simulink model "Puma"  (R2018b)
settings: Solver=VariableStepAuto  StartTime=0.0  StopTime=2  RelTol=1e-3
values from neighbouring files (symbols this model uses):
  Bm = 0.01    [Run.m]
  Kb = 7.5    [Run.m]
  Km = 7.5    [Run.m]
  m1d = m1*d/(h+d)    (= 0.375)    [Run.m]
  m1h = m1*h/(h+d)    (= 1.625)    [Run.m]
  r = 50    [Run.m]
  Ra = 50    [Run.m]
  th1_0 = 0    [Run.m]
  th2_0 = 0    [Run.m]
  th3_0 = 0    [Run.m]
  Va1 = Va    (= 48)    [Run.m]
  Va2 = Va    (= 48)    [Run.m]
  Va3 = Va    (= 48)    [Run.m]
libraries: nesl_utility x13, sm_lib x11
settings Model: Creator=Erfan Etesami  LastModifiedBy=Erfan Etesami

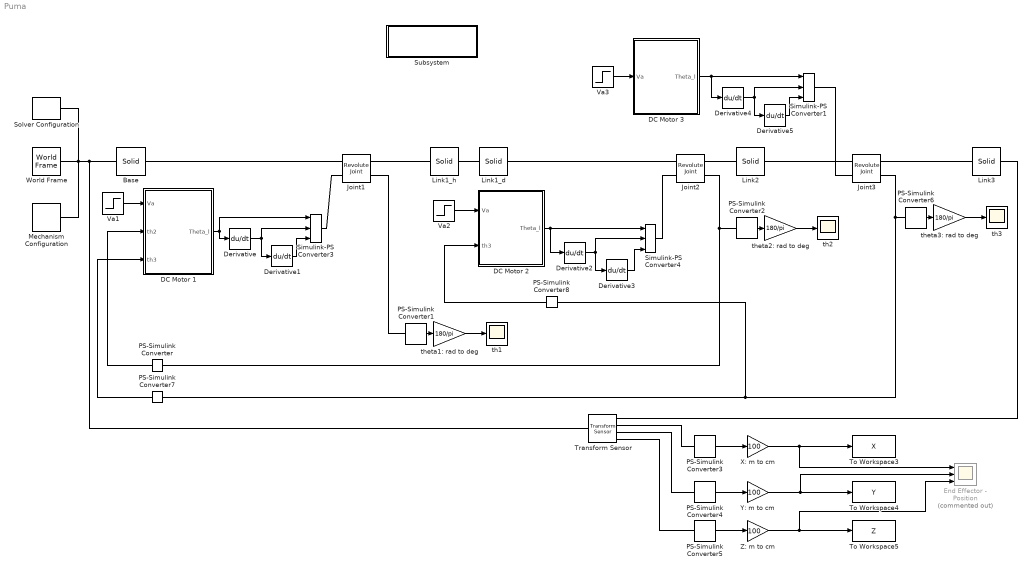
== system Puma ==
  Base : sm_lib/Body Elements/Solid  InertiaType=CalculateFromGeometry  Mass=1  MassUnits=kg  CenterOfMass=[0 0 0]  CenterOfMassUnits=m  MomentsOfInertia=[1 1 1]  MomentsOfInertiaUnits=kg*m^2  ProductsOfInertia=[0 0 0]  ProductsOfInertiaUnits=kg*m^2  BasedOnType=Density  Density=1000  DensityUnits=kg/m^3  DoExposeReferenceFrame=off  SerializedFrames=<Frames><Frame><Id>Frame1</Id><Value><Name>F0</Name><Origin><Source>GeometricFeature</Source><FeatureName>bottom surface</FeatureName></Origin><PrimaryAxis><DefinedDirection>+Y</DefinedDirection><Source>ReferenceFrame</Source><SourceDirection>+Z</SourceDirection><FeatureName></FeatureName></PrimaryAxis><SecondaryAxis><DefinedDirection>+X</DefinedDirection><Source>ReferenceFrame</Source><SourceDirection>+X</SourceDirection><FeatureName></FeatureName></SecondaryAxis></Value></Frame><Frame><Id>Frame2</Id><Value><Name>Ft</Name><Origin><Source>GeometricFeature</Source><FeatureName>bottom surface</FeatureName></Origin><PrimaryAxis><DefinedDirection>+Z</DefinedDirection><Source>ReferenceFrame</Source><SourceDirection>+Z</SourceDirection><FeatureName></FeatureName></PrimaryAxis><SecondaryAxis><DefinedDirection>+X</DefinedDirection><Source>ReferenceFrame</Source><SourceDirection>+X</SourceDirection><FeatureName></FeatureName></SecondaryAxis></Value></Frame></Frames>  GraphicType=FromGeometry  MarkerShape=Sphere  MarkerSize=10  GraphicVisPropType=SimpleVisualProperties  GraphicDiffuseColor=[0.5 0.5 0.5]  GraphicSpecularColor=[0.5 0.5 0.5 1.0]  GraphicAmbientColor=[0.15 0.15 0.15 1.0]  GraphicEmissiveColor=[0.0 0.0 0.0 1.0]  GraphicShininess=75  GraphicOpacity=1.0  GeometryShape=Cylinder  RectangleSize=[1 1]  RectangleSizeUnits=m  BrickDimensions=[1 1 65]  BrickDimensionUnits=cm  CylinderRadius=10  CylinderRadiusUnits=cm  CylinderLength=5  CylinderLengthUnits=cm  SphereRadius=1  SphereRadiusUnits=m  EllipsoidRadii=[1 1 1]  EllipsoidRadiiUnits=m  ExtrusionCrossSection=[1 1; -1 1; -1 -1; 1 -1]  ExtrusionCrossSectionUnits=m  ExtrusionLength=1  ExtrusionLengthUnits=m  PolygonNumSides=3  PolygonOuterRadius=1  PolygonOuterRadiusUnits=m  ExtGeomFileType=STEP  ExtGeomFileUnits=m  RevolutionCrossSection=[1 1; 1 -1; 2 -1; 2 1]  RevolutionCrossSectionUnits=m  RevolutionExtent=Full  RevolutionAngle=180  RevolutionAngleUnits=deg
  DC Motor 1 : Subsystem
  DC Motor 2 : Subsystem
  DC Motor 3 : Subsystem
  Derivative{,1..5} (6 alike) : Derivative
  End Effector - Position : Scope  Commented=on  NumInputPorts=3
  Joint1 : sm_lib/Joints/Revolute Joint  SenseConstraintForce=off  SenseConstraintForceX=off  SenseConstraintForceY=off  SenseConstraintForceZ=off  SenseConstraintTorque=off  SenseConstraintTorqueX=off  SenseConstraintTorqueY=off  SenseConstraintTorqueZ=off  SenseTotalForce=off  SenseTotalForceX=off  SenseTotalForceY=off  SenseTotalForceZ=off  SenseTotalTorque=off  SenseTotalTorqueX=off  SenseTotalTorqueY=off  SenseTotalTorqueZ=off  CompositeWrenchDir=FollowerOnBase  CompositeWrenchFrame=BaseFrame  EquilibriumPosition=0  EquilibriumPositionUnits=deg  SpringStiffness=0  SpringStiffnessUnits=N*m/deg  DampingCoefficient=0  DampingCoefficientUnits=N*m/(deg/s)  TorqueActuationMode=ComputedTorque  MotionActuationMode=InputMotion  SensePosition=on  SenseVelocity=off  SenseAcceleration=off  SenseTorqueForce=off  PositionTargetSpecify=off  PositionTargetPriority=High  PositionTargetValue=0  PositionTargetValueUnits=deg  VelocityTargetSpecify=off  VelocityTargetPriority=High  VelocityTargetValue=0  VelocityTargetValueUnits=deg/s
  Joint2 : sm_lib/Joints/Revolute Joint  SenseConstraintForce=off  SenseConstraintForceX=off  SenseConstraintForceY=off  SenseConstraintForceZ=off  SenseConstraintTorque=off  SenseConstraintTorqueX=off  SenseConstraintTorqueY=off  SenseConstraintTorqueZ=off  SenseTotalForce=off  SenseTotalForceX=off  SenseTotalForceY=off  SenseTotalForceZ=off  SenseTotalTorque=off  SenseTotalTorqueX=off  SenseTotalTorqueY=off  SenseTotalTorqueZ=off  CompositeWrenchDir=FollowerOnBase  CompositeWrenchFrame=BaseFrame  EquilibriumPosition=0  EquilibriumPositionUnits=deg  SpringStiffness=0  SpringStiffnessUnits=N*m/deg  DampingCoefficient=0  DampingCoefficientUnits=N*m/(deg/s)  TorqueActuationMode=ComputedTorque  MotionActuationMode=InputMotion  SensePosition=on  SenseVelocity=off  SenseAcceleration=off  SenseTorqueForce=off  PositionTargetSpecify=off  PositionTargetPriority=High  PositionTargetValue=0  PositionTargetValueUnits=deg  VelocityTargetSpecify=off  VelocityTargetPriority=High  VelocityTargetValue=0  VelocityTargetValueUnits=deg/s
  Joint3 : sm_lib/Joints/Revolute Joint  SenseConstraintForce=off  SenseConstraintForceX=off  SenseConstraintForceY=off  SenseConstraintForceZ=off  SenseConstraintTorque=off  SenseConstraintTorqueX=off  SenseConstraintTorqueY=off  SenseConstraintTorqueZ=off  SenseTotalForce=off  SenseTotalForceX=off  SenseTotalForceY=off  SenseTotalForceZ=off  SenseTotalTorque=off  SenseTotalTorqueX=off  SenseTotalTorqueY=off  SenseTotalTorqueZ=off  CompositeWrenchDir=FollowerOnBase  CompositeWrenchFrame=BaseFrame  EquilibriumPosition=0  EquilibriumPositionUnits=deg  SpringStiffness=0  SpringStiffnessUnits=N*m/deg  DampingCoefficient=0  DampingCoefficientUnits=N*m/(deg/s)  TorqueActuationMode=ComputedTorque  MotionActuationMode=InputMotion  SensePosition=on  SenseVelocity=off  SenseAcceleration=off  SenseTorqueForce=off  PositionTargetSpecify=off  PositionTargetPriority=High  PositionTargetValue=0  PositionTargetValueUnits=deg  VelocityTargetSpecify=off  VelocityTargetPriority=High  VelocityTargetValue=0  VelocityTargetValueUnits=deg/s
  Link1_d : sm_lib/Body Elements/Solid  InertiaType=CalculateFromGeometry  Mass=m1d  MassUnits=kg  CenterOfMass=[0 0 0]  CenterOfMassUnits=m  MomentsOfInertia=[1 1 1]  MomentsOfInertiaUnits=kg*m^2  ProductsOfInertia=[0 0 0]  ProductsOfInertiaUnits=kg*m^2  BasedOnType=Mass  Density=1000  DensityUnits=kg/m^3  DoExposeReferenceFrame=off  SerializedFrames=<Frames><Frame><Id>Frame1</Id><Value><Name>Fm</Name><Origin><Source>GeometricFeature</Source><FeatureName>bottom surface</FeatureName></Origin><PrimaryAxis><DefinedDirection>+Z</DefinedDirection><Source>ReferenceFrame</Source><SourceDirection>+Z</SourceDirection><FeatureName></FeatureName></PrimaryAxis><SecondaryAxis><DefinedDirection>+X</DefinedDirection><Source>ReferenceFrame</Source><SourceDirection>+X</SourceDirection><FeatureName></FeatureName></SecondaryAxis></Value></Frame><Frame><Id>Frame2</Id><Value><Name>F2</Name><Origin><Source>GeometricFeature</Source><FeatureName>top surface</FeatureName></Origin><PrimaryAxis><DefinedDirection>+Z</DefinedDirection><Source>ReferenceFrame</Source><SourceDirection>+Z</SourceDirection><FeatureName></FeatureName></PrimaryAxis><SecondaryAxis><DefinedDirection>+X</DefinedDirection><Source>ReferenceFrame</Source><SourceDirection>+X</SourceDirection><FeatureName></FeatureName></SecondaryAxis></Value></Frame></Frames>  GraphicType=FromGeometry  MarkerShape=Sphere  MarkerSize=10  GraphicVisPropType=SimpleVisualProperties  GraphicDiffuseColor=[1.0 0.0 0.0]  GraphicSpecularColor=[0.5 0.5 0.5 1.0]  GraphicAmbientColor=[0.15 0.15 0.15 1.0]  GraphicEmissiveColor=[0.0 0.0 0.0 1.0]  GraphicShininess=75  GraphicOpacity=1.0  GeometryShape=Cylinder  RectangleSize=[1 1]  RectangleSizeUnits=m  BrickDimensions=[1 1 65]  BrickDimensionUnits=cm  CylinderRadius=R  CylinderRadiusUnits=m  CylinderLength=d  CylinderLengthUnits=m  SphereRadius=1  SphereRadiusUnits=m  EllipsoidRadii=[1 1 1]  EllipsoidRadiiUnits=m  ExtrusionCrossSection=[1 1; -1 1; -1 -1; 1 -1]  ExtrusionCrossSectionUnits=m  ExtrusionLength=1  ExtrusionLengthUnits=m  PolygonNumSides=3  PolygonOuterRadius=1  PolygonOuterRadiusUnits=m  ExtGeomFileType=STEP  ExtGeomFileUnits=m  RevolutionCrossSection=[1 1; 1 -1; 2 -1; 2 1]  RevolutionCrossSectionUnits=m  RevolutionExtent=Full  RevolutionAngle=180  RevolutionAngleUnits=deg
  Link1_h : sm_lib/Body Elements/Solid  InertiaType=CalculateFromGeometry  Mass=m1h  MassUnits=kg  CenterOfMass=[0 0 0]  CenterOfMassUnits=m  MomentsOfInertia=[1 1 1]  MomentsOfInertiaUnits=kg*m^2  ProductsOfInertia=[0 0 0]  ProductsOfInertiaUnits=kg*m^2  BasedOnType=Mass  Density=1000  DensityUnits=kg/m^3  DoExposeReferenceFrame=off  SerializedFrames=<Frames><Frame><Id>Frame1</Id><Value><Name>Ft</Name><Origin><Source>GeometricFeature</Source><FeatureName>bottom surface</FeatureName></Origin><PrimaryAxis><DefinedDirection>+Z</DefinedDirection><Source>ReferenceFrame</Source><SourceDirection>+Z</SourceDirection><FeatureName></FeatureName></PrimaryAxis><SecondaryAxis><DefinedDirection>+X</DefinedDirection><Source>ReferenceFrame</Source><SourceDirection>+X</SourceDirection><FeatureName></FeatureName></SecondaryAxis></Value></Frame><Frame><Id>Frame2</Id><Value><Name>F1</Name><Origin><Source>GeometricFeature</Source><FeatureName>top surface</FeatureName></Origin><PrimaryAxis><DefinedDirection>+Y</DefinedDirection><Source>ReferenceFrame</Source><SourceDirection>+Z</SourceDirection><FeatureName></FeatureName></PrimaryAxis><SecondaryAxis><DefinedDirection>+X</DefinedDirection><Source>ReferenceFrame</Source><SourceDirection>+X</SourceDirection><FeatureName></FeatureName></SecondaryAxis></Value></Frame></Frames>  GraphicType=FromGeometry  MarkerShape=Sphere  MarkerSize=10  GraphicVisPropType=SimpleVisualProperties  GraphicDiffuseColor=[1.0 1.0 0.0]  GraphicSpecularColor=[0.5 0.5 0.5 1.0]  GraphicAmbientColor=[0.15 0.15 0.15 1.0]  GraphicEmissiveColor=[0.0 0.0 0.0 1.0]  GraphicShininess=75  GraphicOpacity=1.0  GeometryShape=Cylinder  RectangleSize=[1 1]  RectangleSizeUnits=m  BrickDimensions=[1 1 65]  BrickDimensionUnits=cm  CylinderRadius=R  CylinderRadiusUnits=m  CylinderLength=h  CylinderLengthUnits=m  SphereRadius=1  SphereRadiusUnits=m  EllipsoidRadii=[1 1 1]  EllipsoidRadiiUnits=m  ExtrusionCrossSection=[1 1; -1 1; -1 -1; 1 -1]  ExtrusionCrossSectionUnits=m  ExtrusionLength=1  ExtrusionLengthUnits=m  PolygonNumSides=3  PolygonOuterRadius=1  PolygonOuterRadiusUnits=m  ExtGeomFileType=STEP  ExtGeomFileUnits=m  RevolutionCrossSection=[1 1; 1 -1; 2 -1; 2 1]  RevolutionCrossSectionUnits=m  RevolutionExtent=Full  RevolutionAngle=180  RevolutionAngleUnits=deg
  Link2 : sm_lib/Body Elements/Solid  InertiaType=CalculateFromGeometry  Mass=4  MassUnits=kg  CenterOfMass=[0 0 0]  CenterOfMassUnits=m  MomentsOfInertia=[1 1 1]  MomentsOfInertiaUnits=kg*m^2  ProductsOfInertia=[0 0 0]  ProductsOfInertiaUnits=kg*m^2  BasedOnType=Mass  Density=1000  DensityUnits=kg/m^3  DoExposeReferenceFrame=off  SerializedFrames=<Frames><Frame><Id>Frame1</Id><Value><Name>F2</Name><Origin><Source>GeometricFeature</Source><FeatureName>bottom surface</FeatureName></Origin><PrimaryAxis><DefinedDirection>+Z</DefinedDirection><Source>ReferenceFrame</Source><SourceDirection>-Y</SourceDirection><FeatureName></FeatureName></PrimaryAxis><SecondaryAxis><DefinedDirection>+X</DefinedDirection><Source>ReferenceFrame</Source><SourceDirection>+Z</SourceDirection><FeatureName></FeatureName></SecondaryAxis></Value></Frame><Frame><Id>Frame2</Id><Value><Name>F3</Name><Origin><Source>GeometricFeature</Source><FeatureName>top surface</FeatureName></Origin><PrimaryAxis><DefinedDirection>+Z</DefinedDirection><Source>ReferenceFrame</Source><SourceDirection>-Y</SourceDirection><FeatureName></FeatureName></PrimaryAxis><SecondaryAxis><DefinedDirection>+X</DefinedDirection><Source>ReferenceFrame</Source><SourceDirection>+Z</SourceDirection><FeatureName></FeatureName></SecondaryAxis></Value></Frame></Frames>  GraphicType=FromGeometry  MarkerShape=Sphere  MarkerSize=10  GraphicVisPropType=SimpleVisualProperties  GraphicDiffuseColor=[1.0 0.2 1.0]  GraphicSpecularColor=[0.5 0.5 0.5 1.0]  GraphicAmbientColor=[0.15 0.15 0.15 1.0]  GraphicEmissiveColor=[0.0 0.0 0.0 1.0]  GraphicShininess=75  GraphicOpacity=1.0  GeometryShape=Cylinder  RectangleSize=[1 1]  RectangleSizeUnits=m  BrickDimensions=[5 5 45]  BrickDimensionUnits=cm  CylinderRadius=R  CylinderRadiusUnits=m  CylinderLength=l1  CylinderLengthUnits=m  SphereRadius=1  SphereRadiusUnits=cm  EllipsoidRadii=[1 1 1]  EllipsoidRadiiUnits=m  ExtrusionCrossSection=[1 1; -1 1; -1 -1; 1 -1]  ExtrusionCrossSectionUnits=m  ExtrusionLength=1  ExtrusionLengthUnits=m  PolygonNumSides=3  PolygonOuterRadius=1  PolygonOuterRadiusUnits=m  ExtGeomFileType=STEP  ExtGeomFileUnits=m  RevolutionCrossSection=[1 1; 1 -1; 2 -1; 2 1]  RevolutionCrossSectionUnits=m  RevolutionExtent=Full  RevolutionAngle=180  RevolutionAngleUnits=deg
  Link3 : sm_lib/Body Elements/Solid  InertiaType=CalculateFromGeometry  Mass=4  MassUnits=kg  CenterOfMass=[0 0 0]  CenterOfMassUnits=m  MomentsOfInertia=[1 1 1]  MomentsOfInertiaUnits=kg*m^2  ProductsOfInertia=[0 0 0]  ProductsOfInertiaUnits=kg*m^2  BasedOnType=Mass  Density=1000  DensityUnits=kg/m^3  DoExposeReferenceFrame=off  SerializedFrames=<Frames><Frame><Id>Frame1</Id><Value><Name>F3</Name><Origin><Source>GeometricFeature</Source><FeatureName>bottom surface</FeatureName></Origin><PrimaryAxis><DefinedDirection>+Z</DefinedDirection><Source>ReferenceFrame</Source><SourceDirection>-Y</SourceDirection><FeatureName></FeatureName></PrimaryAxis><SecondaryAxis><DefinedDirection>+X</DefinedDirection><Source>ReferenceFrame</Source><SourceDirection>+Z</SourceDirection><FeatureName></FeatureName></SecondaryAxis></Value></Frame><Frame><Id>Frame2</Id><Value><Name>F4</Name><Origin><Source>GeometricFeature</Source><FeatureName>top surface</FeatureName></Origin><PrimaryAxis><DefinedDirection>+Z</DefinedDirection><Source>ReferenceFrame</Source><SourceDirection>-Y</SourceDirection><FeatureName></FeatureName></PrimaryAxis><SecondaryAxis><DefinedDirection>+X</DefinedDirection><Source>ReferenceFrame</Source><SourceDirection>+Z</SourceDirection><FeatureName></FeatureName></SecondaryAxis></Value></Frame></Frames>  GraphicType=FromGeometry  MarkerShape=Sphere  MarkerSize=10  GraphicVisPropType=SimpleVisualProperties  GraphicDiffuseColor=[1.0 0.6 0.2]  GraphicSpecularColor=[0.5 0.5 0.5 1.0]  GraphicAmbientColor=[0.15 0.15 0.15 1.0]  GraphicEmissiveColor=[0.0 0.0 0.0 1.0]  GraphicShininess=75  GraphicOpacity=1.0  GeometryShape=Cylinder  RectangleSize=[1 1]  RectangleSizeUnits=m  BrickDimensions=[5 5 55]  BrickDimensionUnits=cm  CylinderRadius=R  CylinderRadiusUnits=m  CylinderLength=l2  CylinderLengthUnits=m  SphereRadius=1  SphereRadiusUnits=m  EllipsoidRadii=[1 1 1]  EllipsoidRadiiUnits=m  ExtrusionCrossSection=[1 1; -1 1; -1 -1; 1 -1]  ExtrusionCrossSectionUnits=m  ExtrusionLength=1  ExtrusionLengthUnits=m  PolygonNumSides=3  PolygonOuterRadius=1  PolygonOuterRadiusUnits=m  ExtGeomFileType=STEP  ExtGeomFileUnits=m  RevolutionCrossSection=[1 1; 1 -1; 2 -1; 2 1]  RevolutionCrossSectionUnits=m  RevolutionExtent=Full  RevolutionAngle=180  RevolutionAngleUnits=deg
  Mechanism Configuration : sm_lib/Utilities/Mechanism Configuration  UniformGravity=Constant  GravityVector=[0 -9.80665 0]  GravityUnits=m/s^2  LinearizationDelta=0.001
  PS-Simulink Converter{,1..8} (9 alike) : nesl_utility/PS-Simulink Converter  PhysicalDomain=network_engine_domain  SubClassName=ps_output  LeftPortType=input  RightPortType=output  PseudoPeriodic=off  Frequencies=[]  Unit=1  AffineConversion=off
  Simulink-PS Converter1 : nesl_utility/Simulink-PS Converter  PhysicalDomain=network_engine_domain  SubClassName=ps_input  LeftPortType=input  RightPortType=output  PseudoPeriodic=off  Frequencies=[]  NoiseDistribution=none  NoiseParameters=[]  Unit=1  AffineConversion=off  FilteringAndDerivatives=provide  SimscapeFilterOrder=1  InputFilterTimeConstant=0.001  UdotUserProvided=2
  Simulink-PS Converter3 : nesl_utility/Simulink-PS Converter  PhysicalDomain=network_engine_domain  SubClassName=ps_input  LeftPortType=input  RightPortType=output  PseudoPeriodic=off  Frequencies=[]  NoiseDistribution=none  NoiseParameters=[]  Unit=1  AffineConversion=off  FilteringAndDerivatives=provide  SimscapeFilterOrder=1  InputFilterTimeConstant=0.001  UdotUserProvided=2
  Simulink-PS Converter4 : nesl_utility/Simulink-PS Converter  PhysicalDomain=network_engine_domain  SubClassName=ps_input  LeftPortType=input  RightPortType=output  PseudoPeriodic=off  Frequencies=[]  NoiseDistribution=none  NoiseParameters=[]  Unit=1  AffineConversion=off  FilteringAndDerivatives=provide  SimscapeFilterOrder=1  InputFilterTimeConstant=0.001  UdotUserProvided=2
  Solver Configuration : nesl_utility/Solver Configuration  PhysicalDomain=network_engine_domain  SubClassName=solver  LeftPortType=input  RightPortType=generic  Tones=[]  Harmonics=[]  SimulateNoise=off  Profile=off  UseLocalSampling=off  EnableSwitchedLinearOptims=on  FrequencyDomain=off  UseCCode=off  RelTol=0.001  AbsTol=1e-06  MinStep=1e-09  ToWorkspace=off  RevertToSquareIcSolve=off  NumHomotopyIterations=100  PhasorMode=off  PhasorModeNumHarmonics=1  DoDC=off  ResidualTolerance=1e-09  UseLocalSolver=off  LocalSolverChoice=NE_BACKWARD_EULER_ADVANCER  LocalSolverSampleTime=0.001  DoFixedCost=off  MaxNonlinIter=3  MaxModeIter=2  LinearAlgebra=Sparse  EquationFormulation=NE_TIME_EF  DelaysMemoryBudget=1024  AutomaticFiltering=on  FilteringTimeConstant=0.001  PartitionStorageMethod=AS_NEEDED  PartitionMemoryBudget=1024
  Subsystem : Subsystem
      settings: OpenFcn=open_system('sm_lib')
      mask Display: disp(sprintf('Open Simscape Multibody\nLibrary'));
  To Workspace3 : ToWorkspace  VariableName=X  SaveFormat=Timeseries  SampleTime=-1
  To Workspace4 : ToWorkspace  VariableName=Y  SaveFormat=Timeseries  SampleTime=-1
  To Workspace5 : ToWorkspace  VariableName=Z  SaveFormat=Timeseries  SampleTime=-1
  Transform Sensor : sm_lib/Frames and Transforms/Transform Sensor  MeasurementFrame=World  SenseAngle=off  SenseAxis=off  SenseAngle1=off  SenseAngle2=off  SenseAngle3=off  SenseQ=off  SenseR=off  SenseOmegaX=off  SenseOmegaY=off  SenseOmegaZ=off  SenseOmega1=off  SenseOmega2=off  SenseOmega3=off  SenseQDot=off  SenseRDot=off  SenseAlphaX=off  SenseAlphaY=off  SenseAlphaZ=off  SenseAlpha1=off  SenseAlpha2=off  SenseAlpha3=off  SenseQDDot=off  SenseRDDot=off  SenseX=on  SenseY=on  SenseZ=on  SenseRad=off  SenseAzim=off  SenseDist=off  SenseInc=off  SenseXDot=off  SenseYDot=off  SenseZDot=off  SenseRadDot=off  SenseAzimDot=off  SenseDistDot=off  SenseIncDot=off  SenseXDDot=off  SenseYDDot=off  SenseZDDot=off  SenseRadDDot=off  SenseAzimDDot=off  SenseDistDDot=off  SenseIncDDot=off
  Va1 : Step  Time=0  After=Va1  SampleTime=0
  Va2 : Step  Time=0  After=Va2  SampleTime=0
  Va3 : Step  Time=0  After=Va3  SampleTime=0
  World Frame : sm_lib/Frames and Transforms/World Frame
  X: m to cm : Gain  Gain=100
  Y: m to cm : Gain  Gain=100
  Z: m to cm : Gain  Gain=100
  th1 : Scope
  th2 : Scope
  th3 : Scope
  theta1: rad to deg : Gain  Gain=180/pi
  theta2: rad to deg : Gain  Gain=180/pi
  theta3: rad to deg : Gain  Gain=180/pi
  wires:
  PS-Simulink Converter5/1 -> Z: m to cm/1
  Y: m to cm/1 -> End Effector - Position/2, To Workspace4/1
  PS-Simulink Converter3/1 -> X: m to cm/1
  PS-Simulink Converter4/1 -> Y: m to cm/1
  Z: m to cm/1 -> End Effector - Position/3, To Workspace5/1
  X: m to cm/1 -> End Effector - Position/1, To Workspace3/1
  Va1/1 -> DC Motor 1/1(Va)
  DC Motor 1/1(Theta_l) -> Simulink-PS Converter3/1, Derivative/1
  Va2/1 -> DC Motor 2/1(Va)
  theta1: rad to deg/1 -> th1/1
  PS-Simulink Converter1/1 -> theta1: rad to deg/1
  PS-Simulink Converter2/1 -> theta2: rad to deg/1
  theta2: rad to deg/1 -> th2/1
  theta3: rad to deg/1 -> th3/1
  PS-Simulink Converter6/1 -> theta3: rad to deg/1
  Derivative1/1 -> Simulink-PS Converter3/3
  Derivative/1 -> Simulink-PS Converter3/2, Derivative1/1
  Derivative2/1 -> Derivative3/1, Simulink-PS Converter4/2
  Derivative3/1 -> Simulink-PS Converter4/3
  Derivative4/1 -> Derivative5/1, Simulink-PS Converter1/2
  Derivative5/1 -> Simulink-PS Converter1/3
  PS-Simulink Converter/1 -> DC Motor 1/2(th2)
  PS-Simulink Converter7/1 -> DC Motor 1/3(th3)
  PS-Simulink Converter8/1 -> DC Motor 2/2(th3)
  DC Motor 2/1(Theta_l) -> Derivative2/1, Simulink-PS Converter4/1
  DC Motor 3/1(Theta_l) -> Derivative4/1, Simulink-PS Converter1/1
  Va3/1 -> DC Motor 3/1(Va)
  connections:
  Base/LConn1 -- Solver Configuration/RConn1 -- Mechanism Configuration/RConn1 -- World Frame/RConn1 -- Transform Sensor/LConn1
  Transform Sensor/RConn1 -- Link3/RConn1
  PS-Simulink Converter4/LConn1 -- Transform Sensor/RConn3
  PS-Simulink Converter3/LConn1 -- Transform Sensor/RConn2
  Joint1/LConn1 -- Base/RConn1
  PS-Simulink Converter5/LConn1 -- Transform Sensor/RConn4
  Joint2/LConn1 -- Link1_d/RConn1
  Link1_d/LConn1 -- Link1_h/RConn1
  Joint3/LConn1 -- Link2/RConn1
  Joint1/RConn1 -- Link1_h/LConn1
  Joint2/RConn1 -- Link2/LConn1
  Joint3/RConn1 -- Link3/LConn1
  PS-Simulink Converter2/LConn1 -- Joint2/RConn2 -- PS-Simulink Converter/LConn1
  Joint3/RConn2 -- PS-Simulink Converter6/LConn1 -- PS-Simulink Converter7/LConn1 -- PS-Simulink Converter8/LConn1
  Joint1/LConn2 -- Simulink-PS Converter3/RConn1
  Joint1/RConn2 -- PS-Simulink Converter1/LConn1
  Joint2/LConn2 -- Simulink-PS Converter4/RConn1
  Joint3/LConn2 -- Simulink-PS Converter1/RConn1

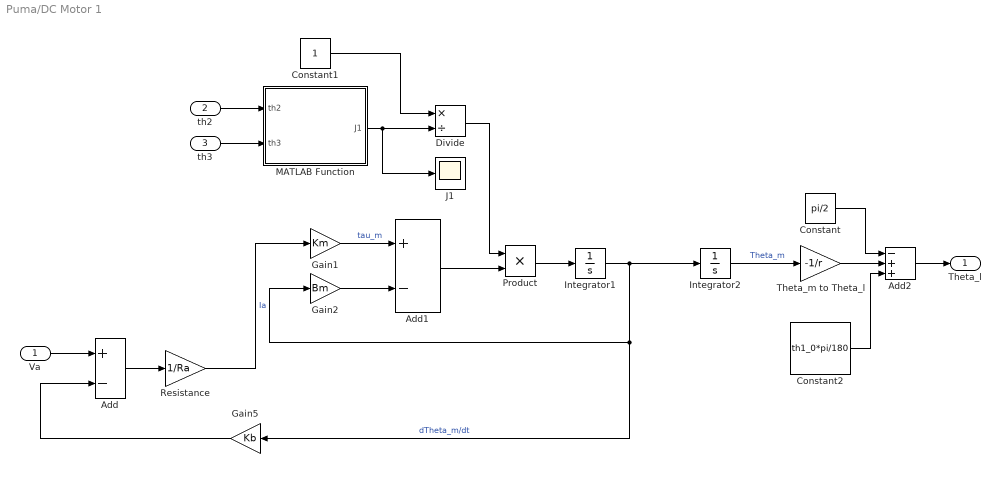
== system Puma/DC Motor 1 ==
  Va : Inport
  th2 : Inport  Port=2
  th3 : Inport  Port=3
  Add : Sum  Inputs=+-
  Add1 : Sum  Inputs=+-
  Add2 : Sum  Inputs=-++
  Constant : Constant  Value=pi/2
  Constant1 : Constant
  Constant2 : Constant  Value=th1_0*pi/180
  Divide : Product  Inputs=*/
  Gain1 : Gain  Gain=Km
  Gain2 : Gain  Gain=Bm
  Gain5 : Gain  Gain=Kb
  Integrator1 : Integrator
  Integrator2 : Integrator
  J1 : Scope
  MATLAB Function : MATLAB Function  TreatAsAtomicUnit=on
  Product : Product
  Resistance : Gain  Gain=1/Ra
  Theta_m to Theta_l : Gain  Gain=-1/r
  Theta_l : Outport
  wires:
  Product/1 -> Integrator1/1
  Gain2/1 -> Add1/2
  Integrator1/1 -> Gain2/1, Gain5/1, Integrator2/1  "dTheta_m/dt"
  Add1/1 -> Product/2
  Resistance/1 -> Gain1/1  "Ia"
  Gain1/1 -> Add1/1  "tau_m"
  Add/1 -> Resistance/1
  Va/1 -> Add/1
  Gain5/1 -> Add/2
  Integrator2/1 -> Theta_m to Theta_l/1  "Theta_m"
  Theta_m to Theta_l/1 -> Add2/2
  Constant/1 -> Add2/1
  Add2/1 -> Theta_l/1
  th2/1 -> MATLAB Function/1(th2)
  th3/1 -> MATLAB Function/2(th3)
  MATLAB Function/1(J1) -> J1/1, Divide/2
  Constant1/1 -> Divide/1
  Divide/1 -> Product/1
  Constant2/1 -> Add2/3

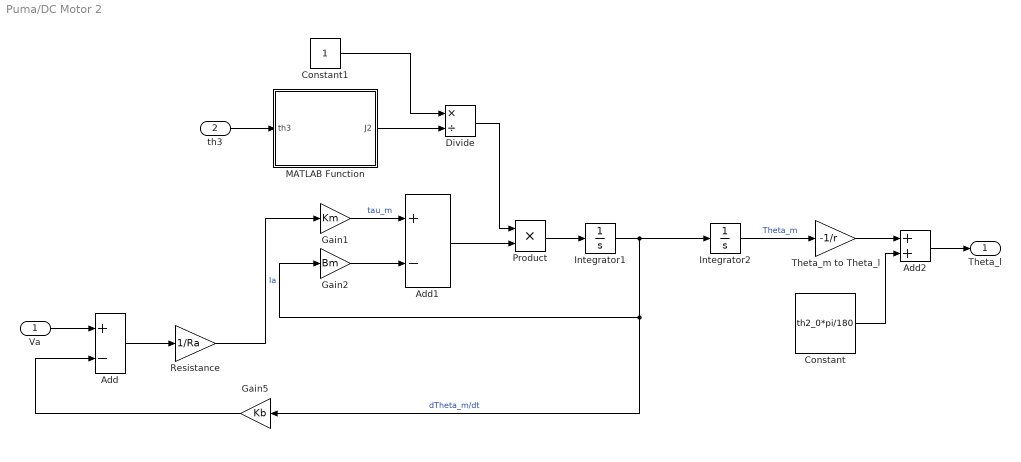
== system Puma/DC Motor 2 ==
  Va : Inport
  th3 : Inport  Port=2
  Add : Sum  Inputs=+-
  Add1 : Sum  Inputs=+-
  Add2 : Sum
  Constant : Constant  Value=th2_0*pi/180
  Constant1 : Constant
  Divide : Product  Inputs=*/
  Gain1 : Gain  Gain=Km
  Gain2 : Gain  Gain=Bm
  Gain5 : Gain  Gain=Kb
  Integrator1 : Integrator
  Integrator2 : Integrator
  MATLAB Function : MATLAB Function  TreatAsAtomicUnit=on
  Product : Product
  Resistance : Gain  Gain=1/Ra
  Theta_m to Theta_l : Gain  Gain=-1/r
  Theta_l : Outport
  wires:
  Divide/1 -> Product/1
  Constant1/1 -> Divide/1
  MATLAB Function/1(J2) -> Divide/2
  th3/1 -> MATLAB Function/1(th3)
  Integrator2/1 -> Theta_m to Theta_l/1  "Theta_m"
  Gain5/1 -> Add/2
  Va/1 -> Add/1
  Add/1 -> Resistance/1
  Gain1/1 -> Add1/1  "tau_m"
  Resistance/1 -> Gain1/1  "Ia"
  Add1/1 -> Product/2
  Integrator1/1 -> Integrator2/1, Gain5/1, Gain2/1  "dTheta_m/dt"
  Gain2/1 -> Add1/2
  Product/1 -> Integrator1/1
  Add2/1 -> Theta_l/1
  Theta_m to Theta_l/1 -> Add2/1
  Constant/1 -> Add2/2

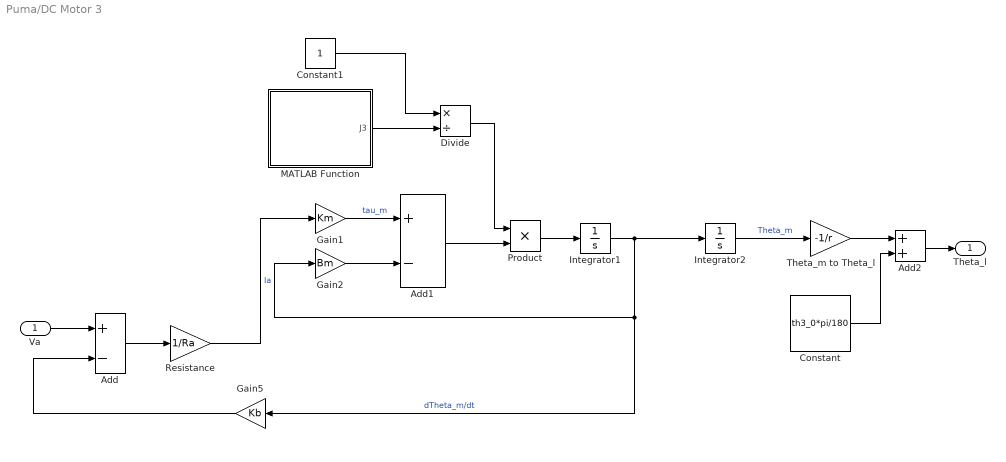
== system Puma/DC Motor 3 ==
  Va : Inport
  Add : Sum  Inputs=+-
  Add1 : Sum  Inputs=+-
  Add2 : Sum
  Constant : Constant  Value=th3_0*pi/180
  Constant1 : Constant
  Divide : Product  Inputs=*/
  Gain1 : Gain  Gain=Km
  Gain2 : Gain  Gain=Bm
  Gain5 : Gain  Gain=Kb
  Integrator1 : Integrator
  Integrator2 : Integrator
  MATLAB Function : MATLAB Function  TreatAsAtomicUnit=on
  Product : Product
  Resistance : Gain  Gain=1/Ra
  Theta_m to Theta_l : Gain  Gain=-1/r
  Theta_l : Outport
  wires:
  Product/1 -> Integrator1/1
  Gain2/1 -> Add1/2
  Integrator1/1 -> Gain2/1, Gain5/1, Integrator2/1  "dTheta_m/dt"
  Add1/1 -> Product/2
  Resistance/1 -> Gain1/1  "Ia"
  Gain1/1 -> Add1/1  "tau_m"
  Add/1 -> Resistance/1
  Va/1 -> Add/1
  Gain5/1 -> Add/2
  Integrator2/1 -> Theta_m to Theta_l/1  "Theta_m"
  MATLAB Function/1(J3) -> Divide/2
  Constant1/1 -> Divide/1
  Divide/1 -> Product/1
  Theta_m to Theta_l/1 -> Add2/1
  Add2/1 -> Theta_l/1
  Constant/1 -> Add2/2

== system Puma/Subsystem ==

== matlab function Puma/DC Motor 2/MATLAB Function ==
  data: J2 output; th3 input
function J2 = calcJ2(th3)
l1 = 45/100;    % m
l2 = 55/100;    % m
m2 = 4; % Kg
m3 = 4; % Kg
r = 50;     % Gear Ratio
Jm = 0.1;   % Kg.m^2
Jg = 0.05;  % Kg.m^2

l2mc = l2*cos(th3);
l2ms = l2*sin(th3);

Jl2 = (1/12)*m2*(l1^2) + m2*((l1/2)^2) +...
      (1/12)*m3*(l2^2) + m3*((l2mc/2 + l1)^2 + (l2ms/2)^2);
 
J2 = Jm + Jg + Jl2/(r^2);
end

== matlab function Puma/DC Motor 1/MATLAB Function ==
  data: th2 input; J1 output; th3 input
function J1 = calcJ1(th2, th3)
d = 15/100;     % m
h = 65/100;     % m
l1 = 45/100;    % m
l2 = 55/100;    % m
m1 = 2; % Kg
m1d = m1*d/(h+d);   % Part d
m2 = 4; % Kg
m3 = 4; % Kg
r = 50;     % Gear Ratio
Jm = 0.1;   % Kg.m^2
Jg = 0.05;  % Kg.m^2

l1m = l1*cos(th2);
l2m = l2*cos(th2+th3);

Jl1 = (1/12)*m1d*(d^2) + m1d*((d/2)^2) +...
      (1/12)*m2*(l1m^2) + m2*((l1m/2)^2 + d^2) +...
      (1/12)*m3*(l2m^2) + m3*((l2m/2 + l1m)^2 + d^2);
  
J1 = Jm + Jg + Jl1/(r^2);
end

== matlab function Puma/DC Motor 3/MATLAB Function ==
  data: J3 output
function J3 = calcJ3()
l2 = 55/100;    % m
m3 = 4; % Kg
r = 50;     % Gear Ratio
Jm = 0.1;   % Kg.m^2
Jg = 0.05;  % Kg.m^2

Jl3 = (1/12)*m3*(l2^2) + m3*((l2/2)^2);
  
J3 = Jm + Jg + Jl3/(r^2);
end
